simulink model "Nominal_design_step_validation"  (R2024b)
settings: Solver=VariableStepAuto  StartTime=0.0  StopTime=45  FixedStep=0.001  RelTol=1e-3
undefined symbols (not defined in the file): degs2rpm, drv, gbox, K, mld, mot, Nu, Nx, rads2rpm, rdp, rpm2rads, sens, Ts, u_bar_max
settings Model: Creator=Enrico  LastModifiedBy=Enrico 2
settings DataIOCC: ReturnWorkspaceOutputsName=out_black_box

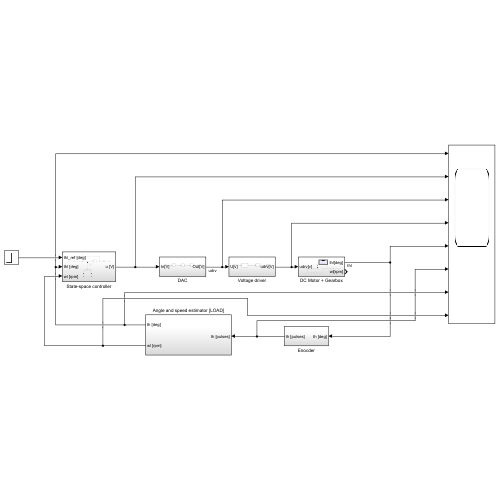
[thumbnail: Simulink's stored preview of the top-level diagram]
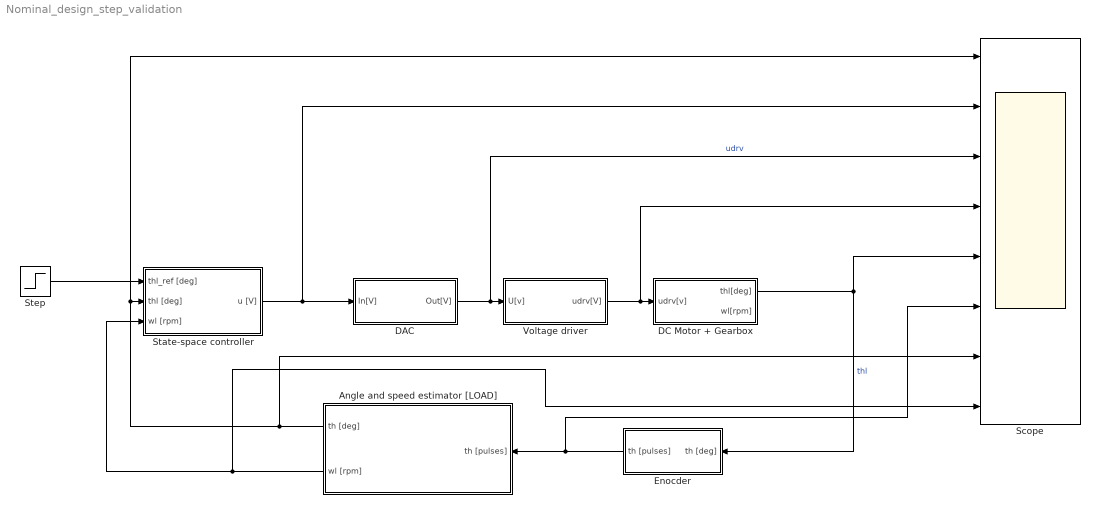
== system Nominal_design_step_validation ==
  Angle and speed estimator [LOAD] : Subsystem
  DAC : Subsystem
  DC Motor + Gearbox : Subsystem
  Enocder : Subsystem
  Scope : Scope  NumInputPorts=8
  State-space controller : Subsystem
  Step : Step  SampleTime=0
  Voltage driver : Subsystem
  wires:
  Step/1 -> State-space controller/1(thl_ref [deg])
  Angle and speed estimator [LOAD]/1(th [deg]) -> Scope/1, State-space controller/2(thl [deg]), Scope/7
  Angle and speed estimator [LOAD]/2(wl [rpm]) -> State-space controller/3(wl [rpm]), Scope/8
  State-space controller/1(u [V]) -> DAC/1(In[V]), Scope/2
  Enocder/1(th [pulses]) -> Scope/6, Angle and speed estimator [LOAD]/1(th [pulses])
  DC Motor + Gearbox/1(thl[deg]) -> Enocder/1(th [deg]), Scope/5  "thl"
  DAC/1(Out[V]) -> Scope/3, Voltage driver/1(U[v])  "udrv"
  Voltage driver/1(udrv[V]) -> Scope/4, DC Motor + Gearbox/1(udrv[v])

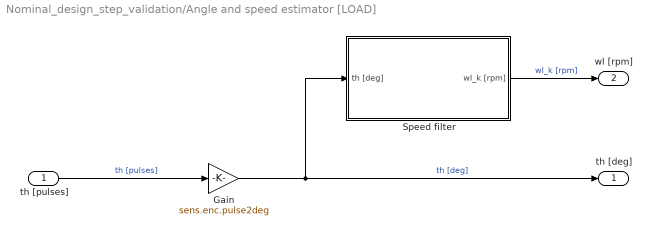
== system Nominal_design_step_validation/Angle and speed estimator [LOAD] ==
  th [pulses] : Inport
  Gain : Gain  Gain=sens.enc.pulse2deg
  Speed filter : Subsystem
  th [deg] : Outport
  wl [rpm] : Outport  Port=2
  wires:
  Speed filter/1(wl_k [rpm]) -> wl [rpm]/1  "wl_k [rpm]"
  th [pulses]/1 -> Gain/1  "th [pulses]"
  Gain/1 -> Speed filter/1(th [deg]), th [deg]/1  "th [deg]"

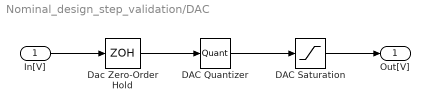
== system Nominal_design_step_validation/DAC ==
  In[V] : Inport
  DAC Quantizer : Quantizer  QuantizationInterval=20/(2^16-1)
  DAC Saturation : Saturate  UpperLimit=10  LowerLimit=-10
  Dac Zero-Order Hold : ZeroOrderHold  SampleTime=Ts
  Out[V] : Outport
  wires:
  In[V]/1 -> Dac Zero-Order Hold/1
  DAC Saturation/1 -> Out[V]/1
  DAC Quantizer/1 -> DAC Saturation/1
  Dac Zero-Order Hold/1 -> DAC Quantizer/1

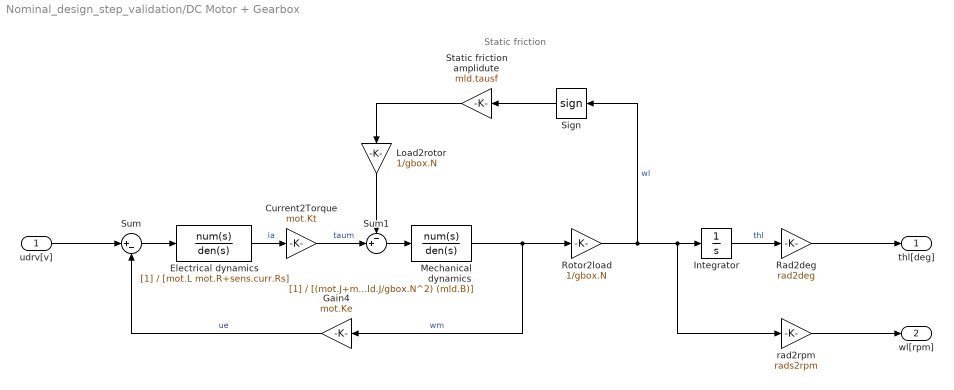
== system Nominal_design_step_validation/DC Motor + Gearbox ==
  note: Static friction
  udrv[v] : Inport
  " Sign" : Signum  ZeroCross=off
  Current2Torque : Gain  Gain=mot.Kt
  Electrical dynamics : TransferFcn  Denominator=[mot.L mot.R+sens.curr.Rs]
  Gain4 : Gain  Gain=mot.Ke
  Integrator : Integrator
  Load2rotor : Gain  Gain=1/gbox.N
  Mechanical dynamics : TransferFcn  Denominator=[(mot.J+mld.J/gbox.N^2) (mld.B)]
  Rad2deg : Gain  Gain=rad2deg
  Rotor2load : Gain  Gain=1/gbox.N
  Static friction amplidute : Gain  Gain=mld.tausf
  Sum : Sum  Inputs=|+-
  Sum1 : Sum  Inputs=-+|
  rad2rpm : Gain  Gain=rads2rpm
  thl[deg] : Outport
  wl[rpm] : Outport  Port=2
  wires:
  udrv[v]/1 -> Sum/1
  Sum/1 -> Electrical dynamics/1
  Electrical dynamics/1 -> Current2Torque/1  "ia"
  Current2Torque/1 -> Sum1/2  "taum"
  Load2rotor/1 -> Sum1/1
  " Sign"/1 -> Static friction amplidute/1
  Static friction amplidute/1 -> Load2rotor/1
  Sum1/1 -> Mechanical dynamics/1
  Mechanical dynamics/1 -> Gain4/1, Rotor2load/1  "wm"
  Gain4/1 -> Sum/2  "ue"
  Rad2deg/1 -> thl[deg]/1
  rad2rpm/1 -> wl[rpm]/1
  Integrator/1 -> Rad2deg/1  "thl"
  Rotor2load/1 -> " Sign"/1, rad2rpm/1, Integrator/1  "wl"

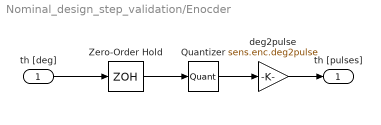
== system Nominal_design_step_validation/Enocder ==
  th [deg] : Inport
  Quantizer : Quantizer  QuantizationInterval=sens.enc.pulse2deg
  Zero-Order Hold : ZeroOrderHold  SampleTime=Ts
  deg2pulse : Gain  Gain=sens.enc.deg2pulse
  th [pulses] : Outport
  wires:
  Quantizer/1 -> deg2pulse/1
  th [deg]/1 -> Zero-Order Hold/1
  Zero-Order Hold/1 -> Quantizer/1
  deg2pulse/1 -> th [pulses]/1

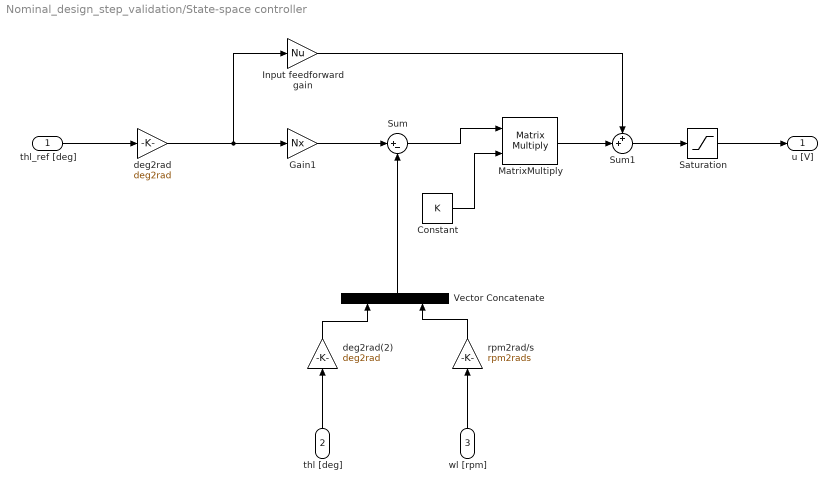
== system Nominal_design_step_validation/State-space controller ==
  thl_ref [deg] : Inport
  thl [deg] : Inport  Port=2
  wl [rpm] : Inport  Port=3
  Constant : Constant  Value=K
  Gain1 : Gain  Gain=Nx
  Input feedforward gain : Gain  Gain=Nu
  MatrixMultiply : Product  Multiplication=Matrix(*)
  Saturation : Saturate  UpperLimit=u_bar_max  LowerLimit=-u_bar_max
  Sum : Sum  Inputs=|+-
  Sum1 : Sum  Inputs=++|
  Vector Concatenate : Concatenate
  deg2rad : Gain  Gain=deg2rad
  deg2rad(2) : Gain  Gain=deg2rad
  rpm2rad/s : Gain  Gain=rpm2rads
  u [V] : Outport
  wires:
  rpm2rad/s/1 -> Vector Concatenate/2
  Gain1/1 -> Sum/1
  Sum1/1 -> Saturation/1
  thl [deg]/1 -> deg2rad(2)/1
  deg2rad/1 -> Input feedforward gain/1, Gain1/1
  deg2rad(2)/1 -> Vector Concatenate/1
  thl_ref [deg]/1 -> deg2rad/1
  wl [rpm]/1 -> rpm2rad/s/1
  Input feedforward gain/1 -> Sum1/1
  Vector Concatenate/1 -> Sum/2
  Saturation/1 -> u [V]/1
  MatrixMultiply/1 -> Sum1/2
  Sum/1 -> MatrixMultiply/1
  Constant/1 -> MatrixMultiply/2

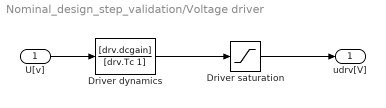
== system Nominal_design_step_validation/Voltage driver ==
  U[v] : Inport
  Driver dynamics : TransferFcn  Numerator=[drv.dcgain]  Denominator=[drv.Tc 1]
  Driver saturation : Saturate  UpperLimit=12  LowerLimit=-12
  udrv[V] : Outport
  wires:
  U[v]/1 -> Driver dynamics/1
  Driver dynamics/1 -> Driver saturation/1
  Driver saturation/1 -> udrv[V]/1

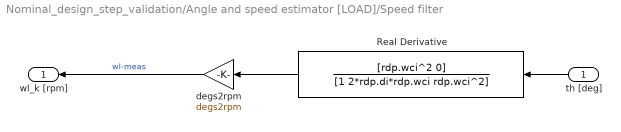
== system Nominal_design_step_validation/Angle and speed estimator [LOAD]/Speed filter ==
  th [deg] : Inport
  Real Derivative : TransferFcn  Numerator=[rdp.wci^2 0]  Denominator=[1 2*rdp.di*rdp.wci rdp.wci^2]
  degs2rpm : Gain  Gain=degs2rpm
  wl_k [rpm] : Outport
  wires:
  th [deg]/1 -> Real Derivative/1
  degs2rpm/1 -> wl_k [rpm]/1  "wl-meas"
  Real Derivative/1 -> degs2rpm/1
